simulink model "F3_Trajectory"  (R2020a)
settings: Solver=VariableStepAuto  StartTime=0.0  StopTime=10.0  RelTol=1e-3
libraries: simulink x7
settings Model: Creator=xeezy  LastModifiedBy=axelzedigh

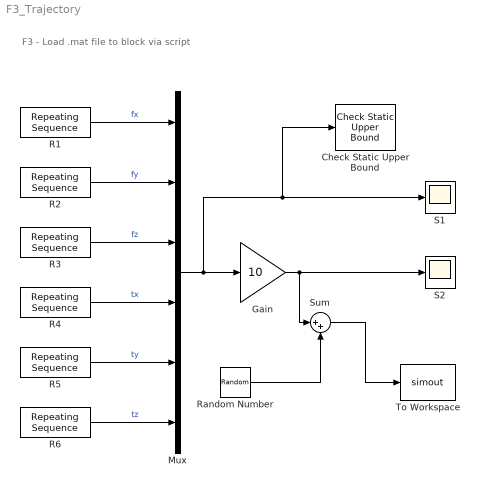
== system F3_Trajectory ==
  note: F3 - Load .mat file to block via script
  Check Static Upper Bound : simulink/Model Verification/Check Static  Upper Bound  Description=u <= 500  max=500  max_included=on  enabled=on  stopWhenAssertionFail=off  export=off  icon=text
      settings: SourceProductBaseCode=SL
  Gain : Gain  Gain=10
  Mux : Mux  Inputs=6
  R1 : simulink/Sources/Repeating Sequence  rep_seq_t=TIME  rep_seq_y=FX
  R2 : simulink/Sources/Repeating Sequence  rep_seq_t=TIME  rep_seq_y=FY
  R3 : simulink/Sources/Repeating Sequence  rep_seq_t=TIME  rep_seq_y=FZ
  R4 : simulink/Sources/Repeating Sequence  rep_seq_t=TIME  rep_seq_y=MX
  R5 : simulink/Sources/Repeating Sequence  rep_seq_t=TIME  rep_seq_y=MY
  R6 : simulink/Sources/Repeating Sequence  rep_seq_t=TIME  rep_seq_y=MZ
  Random Number : RandomNumber  Mean=80  SampleTime=0.1
  S1 : Scope
  S2 : Scope
  Sum : Sum  Inputs=|++
  To Workspace : ToWorkspace  VariableName=simout  SaveFormat=Structure With Time  SampleTime=-1
  wires:
  R1/1 -> Mux/1  "fx"
  R6/1 -> Mux/6  "tz"
  R5/1 -> Mux/5  "ty"
  R4/1 -> Mux/4  "tx"
  R3/1 -> Mux/3  "fz"
  R2/1 -> Mux/2  "fy"
  Mux/1 -> Check Static Upper Bound/1, S1/1, Gain/1
  Gain/1 -> Sum/1, S2/1
  Random Number/1 -> Sum/2
  Sum/1 -> To Workspace/1
